simulink model "human_approval_gate"  (R2026a)
settings: Solver=FixedStepDiscrete  StopTime=1
settings Model: Creator=Nouran Ismail  LastModifiedBy=Nouran Ismail

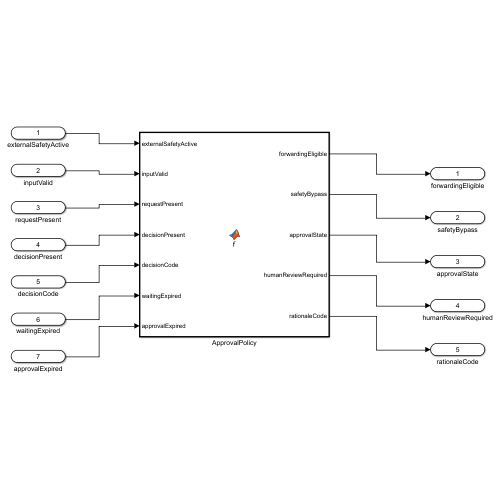
[thumbnail: Simulink's stored preview of the top-level diagram]
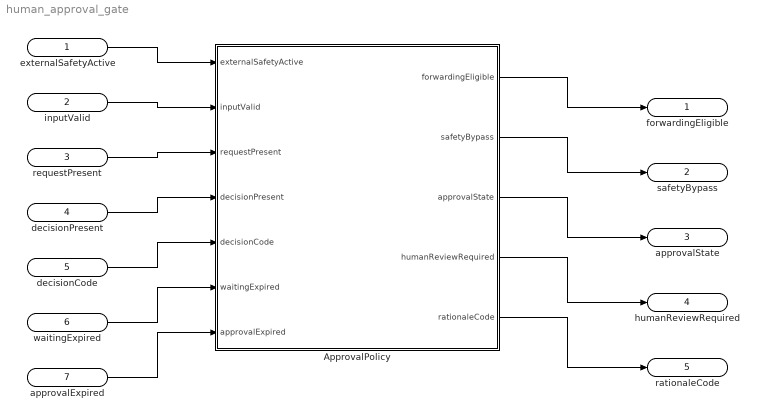
== system human_approval_gate ==
  externalSafetyActive : Inport  OutDataTypeStr=boolean
  inputValid : Inport  Port=2  OutDataTypeStr=boolean
  requestPresent : Inport  Port=3  OutDataTypeStr=boolean
  decisionPresent : Inport  Port=4  OutDataTypeStr=boolean
  decisionCode : Inport  Port=5  OutDataTypeStr=uint8
  waitingExpired : Inport  Port=6  OutDataTypeStr=boolean
  approvalExpired : Inport  Port=7  OutDataTypeStr=boolean
  ApprovalPolicy : MATLAB Function  TreatAsAtomicUnit=on
  forwardingEligible : Outport
  safetyBypass : Outport  Port=2
  approvalState : Outport  Port=3
  humanReviewRequired : Outport  Port=4
  rationaleCode : Outport  Port=5
  wires:
  externalSafetyActive/1 -> ApprovalPolicy/1(externalSafetyActive)
  inputValid/1 -> ApprovalPolicy/2(inputValid)
  requestPresent/1 -> ApprovalPolicy/3(requestPresent)
  decisionPresent/1 -> ApprovalPolicy/4(decisionPresent)
  decisionCode/1 -> ApprovalPolicy/5(decisionCode)
  waitingExpired/1 -> ApprovalPolicy/6(waitingExpired)
  approvalExpired/1 -> ApprovalPolicy/7(approvalExpired)
  ApprovalPolicy/1(forwardingEligible) -> forwardingEligible/1
  ApprovalPolicy/2(safetyBypass) -> safetyBypass/1
  ApprovalPolicy/3(approvalState) -> approvalState/1
  ApprovalPolicy/4(humanReviewRequired) -> humanReviewRequired/1
  ApprovalPolicy/5(rationaleCode) -> rationaleCode/1

== matlab function human_approval_gate/ApprovalPolicy ==
  data: externalSafetyActive input; forwardingEligible output; inputValid input; requestPresent input; decisionPresent input; decisionCode input; waitingExpired input; approvalExpired input; safetyBypass output; approvalState output; humanReviewRequired output; rationaleCode output
function [forwardingEligible,safetyBypass,approvalState,humanReviewRequired,rationaleCode] = f(externalSafetyActive,inputValid,requestPresent,decisionPresent,decisionCode,waitingExpired,approvalExpired)
forwardingEligible=false;
safetyBypass=false;
approvalState=uint8(0);
humanReviewRequired=true;
rationaleCode=uint16(21);
if externalSafetyActive
    safetyBypass=true;
    rationaleCode=uint16(20);
    return;
end
if ~inputValid
    return;
end
if ~requestPresent
    rationaleCode=uint16(22);
    return;
end
if ~decisionPresent
    rationaleCode=uint16(23);
    return;
end
if decisionCode==uint8(0)
    approvalState=uint8(1);
    if waitingExpired
        approvalState=uint8(4);
        rationaleCode=uint16(27);
    else
        rationaleCode=uint16(24);
    end
elseif decisionCode==uint8(3)
    approvalState=uint8(2);
    if waitingExpired
        approvalState=uint8(4);
        rationaleCode=uint16(27);
    else
        rationaleCode=uint16(25);
    end
elseif decisionCode==uint8(2)
    approvalState=uint8(3);
    rationaleCode=uint16(26);
elseif decisionCode==uint8(4)
    approvalState=uint8(4);
    rationaleCode=uint16(28);
elseif decisionCode==uint8(1)
    if approvalExpired
        approvalState=uint8(4);
        rationaleCode=uint16(28);
    else
        approvalState=uint8(5);
        rationaleCode=uint16(29);
        forwardingEligible=true;
        humanReviewRequired=false;
    end
end
end
